simulink model "OFDM_RF_comms_link"  (R2023a)
settings: Solver=FixedStepAuto  StartTime=0.0  StopTime=Tstep*ofdmSymLen*6  RelTol=1e-3
PreLoadFcn:
  | % 100 MHz scenario
  | scs = 30e3;
  | fftLength = 4096;
  | NSubcarriers = 3276;
  | cpLength = 288;
  | windowLength = 20;
  | 
  | nGuardBandCarrier = fftLength - NSubcarriers;
  | ofdmSymLen = fftLength+cpLength;
  | overSamplingRate = 7;
  | filterLength = 6*70;
  | 
  | BW = scs*fftLength;                       %  Signal BW
  | Tstep = 1/BW;                   %  Simulation BW BB
  | RF = 3.7e9;                       %  RF center frequency
  | IF = 500e6;                          % IF frequency
  | dataRatePA = 1/BW;  % PA characterization sample time
  | N = nGuardBandCarrier/2;
  | HPF_cutoff = RF - 500e6;
  | 
  | bw = 100e6;
  | [txWaveform, sampleRate] = helperPACharGenerateOFDM(bw);
  | 
  | dataFileName = sprintf("helperPACharSavedData%dMHz",bw/1e6);
  | load(dataFileName,"results")
  | paInput = results.InputWaveform;
  | paOutput = results.OutputWaveform;
  | modType = 'memPoly';
  | memLen = 5;
  | degLen = 5;
  | halfDataPts = round(length(paInput)/2);
  | origState = warning;
  | warning('off', 'MATLAB:rankDeficientMatrix')
  | paModelMemPoly = double(helperPACharMemPolyModel('coefficientFinder', ...
  |   paInput(1:halfDataPts),paOutput(1:halfDataPts),memLen,degLen,modType));
  | warning(origState);
  | 
  | gain = results.LinearGain;
  | scaleFactor = double(max(abs(paOutput))/max(abs(txWaveform))/gain);
undefined symbols (not defined in the file or in its folder): QAM, rational, S, sparameters
libraries: simrfV2elements x17, simrfV2util1 x5, simrfV2_lib x3, commofdm x2, dspstat3 x2, commrfcorlib x2, commrandsrc3 x1, commdigbbndam3 x1, simrfV2junction1 x1, simrfV2sources1 x1, commutil2 x1, simrfV2systems x1
Description:
  | Power Amplifier Characterization with DPD for Reduced Signal Distortion
settings Model: SimulationMode=accelerator  Creator=The MathWorks, Inc.  LastModifiedBy=pradnyapatil
settings SolverCC: ZeroCrossAlgorithm=Adaptive  AlgebraicLoopSolver=TrustRegion
settings DataIOCC: LimitDataPoints=on  SaveFormat=Array  SaveOutput=off  SignalLogging=off  DSMLogging=off  SaveTime=off  ReturnWorkspaceOutputs=off
settings OptimizationCC: BlockReduction=off  BooleanDataType=off  ReuseModelBlockBuffer=off  LifeSpan=inf
settings DebuggingCC: SaveWithParameterizedLinksMsg=none  UnderspecifiedInitializationDetection=Classic  MergeDetectMultiDrivingBlocksExec=none  SignalResolutionControl=TryResolveAllWithWarning  UnconnectedInputMsg=warning  UnconnectedOutputMsg=warning  UnconnectedLineMsg=warning  AllowSymbolicDim=off  SFUnexpectedBacktrackingDiag=warning  SFNoUnconditionalDefaultTransitionDiag=warning  SFExecutionAtInitializationDiag=none  ArithmeticOperatorsInVariantConditions=warning
settings HardwareCC: ProdBitPerPointer=32  ProdBitPerSizeT=32  ProdBitPerPtrDiffT=32  ProdLargestAtomicFloat=None  ProdIntDivRoundTo=Undefined  ProdEndianess=Unspecified  ProdWordSize=32  ProdHWDeviceType=32-bit Generic  TargetBitPerLong=64  TargetBitPerPointer=64  TargetBitPerSizeT=64  TargetBitPerPtrDiffT=64  TargetLongLongMode=on  TargetIntDivRoundTo=Zero  TargetEndianess=LittleEndian  TargetWordSize=64  TargetHWDeviceType=MATLAB Host  ProdEqTarget=off
settings ModelReferenceCC: EnableRefExpFcnMdlSchedulingChecks=on  PropagateSignalLabelsOutOfModel=off
settings SFSimCC: SimUseLocalCustomCode=off
settings RTWCC: RTWUseLocalCustomCode=off  BuildConfiguration=Faster Runs  DLArmComputeVersion=19.05
settings CodeAppCC: StateflowObjectComments=on
settings GRTTargetCC: TargetLangStandard=C89/C90 (ANSI)
settings ConfigComp: CovMetricSettings=dw  CovSaveCumulativeToWorkspaceVar=on  CovSaveSingleToWorkspaceVar=on  CovExternalEMLEnable=off
settings SimscapeCC: SimscapeNormalizeSystem=off

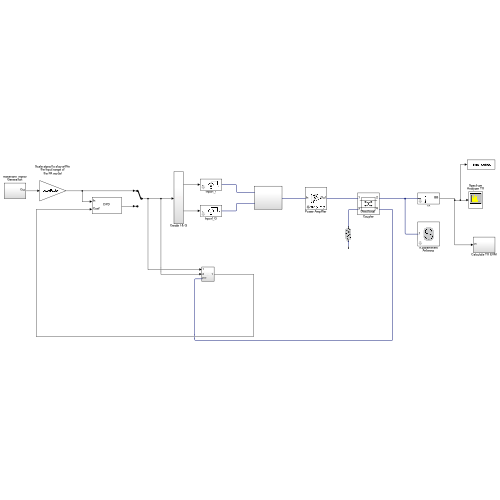
[thumbnail: Simulink's stored preview of the top-level diagram]
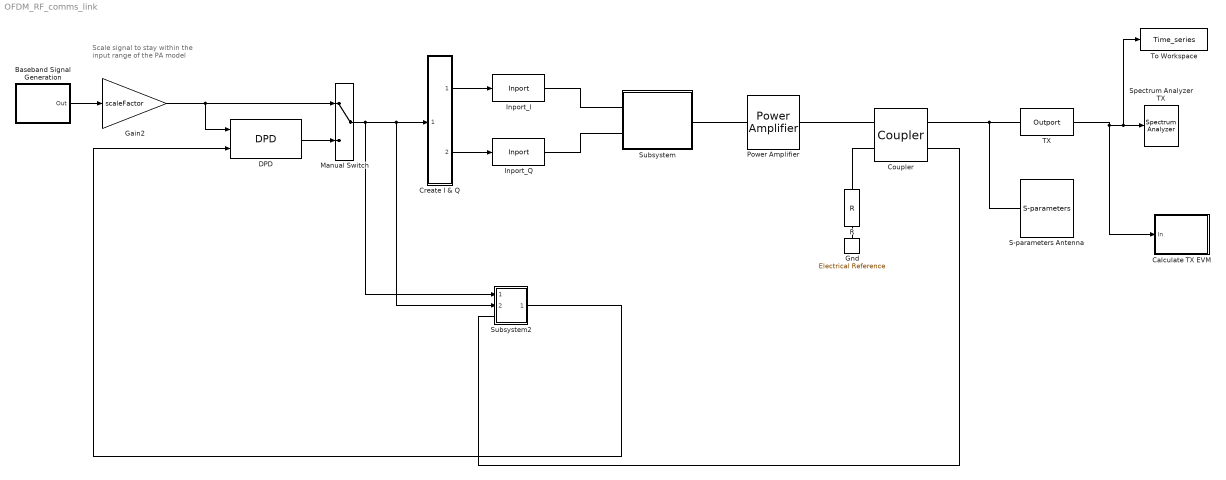
== system OFDM_RF_comms_link ==
  note: Scale signal to stay within
      | the input range of
      | the PA model
  Baseband Signal Generation : Subsystem
  Calculate TX EVM : Subsystem
  Coupler : simrfV2junction1/Coupler  classname=couplers  DataSource=Network-parameters  NumPorts=4  DeviceCirculator=Circulator clockwise  DeviceDivider=T power divider  DeviceCoupler=Directional coupler  Paramtype=S-parameters  Sparam=[0 0 1; 1 0 0; 0 1 0]  SparamFreq=1e9 Hz  SparamZ0=50  Phase12=0  Phase33=0  Alpha=0  NumberDividerOutports=2  Coupling=55  Directivity=inf  InsertionLoss=0.0001  ReturnLoss=inf  InternalGrounding=on  SparamRepresentation=Frequency domain  FitOpt=Share all poles  FitTol=-40  MaxPoles=48
  Create I & Q : Subsystem
  DPD : commrfcorlib/DPD  PolynomialType=Memory polynomial  CoefficientSource=Input port  Coefficients=complex([1 0 0 0 0; 0 0 0 0 0; 0 0 0 0 0])  SimulateUsing=Interpreted execution
  Gain2 : Gain  Gain=scaleFactor
  Gnd : simrfV2_lib/Elements/Electrical Reference
      settings: InternalSimscapePortConfiguration="{\"Bottom\":[],\"Left\":[{\"id\":\"V\",\"label\":\"\",\"type\":\"foundation.rf.circuitenvelope\"}],\"Right\":[],\"Top\":[]}"
  Inport_I : simrfV2util1/Inport  SimulinkInputSignalType=Ideal voltage  CarrierFreq=0 Hz  ZS=0  UseSqWave=off  NumCoeff=10  Bias=0  DutyCyc=50  InternalGrounding=on
  Inport_Q : simrfV2util1/Inport  SimulinkInputSignalType=Ideal voltage  CarrierFreq=0 Hz  ZS=0  UseSqWave=off  NumCoeff=10  Bias=0  DutyCyc=50  InternalGrounding=on
  Manual Switch : ManualSwitch
  Power Amplifier : simrfV2elements/Power Amplifier  classname=poweramp  ModelType=Memory polynomial  CoeffMatrix=paModelMemPoly  UnitDelay=dataRatePA/overSamplingRate  Rin=50  Rout=50  InternalGrounding=on
  R : simrfV2elements/R  classname=resistor  Resistance=50 Ohm  AddNoise=on
  S-parameters Antenna : simrfV2elements/S-parameters  classname=sparam_element  DataSource=Data file  File=antenna_dpdexample.s1p  isNetworkObj=off  NetworkObject=sparameters('default.s2p')  Paramtype=S-parameters  Sparam=[0 0;1 0]  SparamFreq=1e9 Hz  SparamZ0=50  isRationalObj=off  RationalObject=rational('default.s2p')  Residues=0  Poles=0  DF={0 0; 1 0}  FitOpt=Fit individually  FitTol=-40  MaxPoles=48  SourceFreq=Extracted from data source  PlotFreq=[1e9:1e6:3e9] Hz  PlotType=X-Y plane  YParam1=S(1,1)  YFormat1=Magnitude (dB)  YParam2=None  YFormat2=Magnitude (dB)  YOption=Linear  XOption=Linear  AddNoise=on  InternalGrounding=on  SparamRepresentation=Frequency domain  AutoImpulseLength=on  ImpulseLength=1e-10 s  MagModeling=off  CacheLevel=0
  Spectrum Analyzer TX : SpectrumAnalyzer  WindowPosition=[286.000000,108.000000,865.000000,471.000000,]  ScopeFrameLocation=window  Method=Welch  SampleRate=860160000  AxesScaling=Manual  Span=1843200000  StartFrequency=-921600000  StopFrequency=921600000  FrequencyResolutionMethod=Window length  WindowLength=8192  AveragingMethod=Running  SpectralAverages=4  ReferenceLoad=50  YLimits=[-42.635393903054115583 22.757787926364073883]  DefaultConfigurationName=spbscopes.SpectrumAnalyzerBlockCfg  IsFrequencyInputMode=0  FrequencyVectorPort=0  FrequencyVectorFromPort=0  FrequencyInputRBWPort=0  FrequencyInputRBWFromPort=0
  Subsystem : Subsystem
  Subsystem2 : Subsystem
  TX : simrfV2util1/Outport  SensorType=Ideal voltage  OutputFormat=Complex Baseband  CarrierFreq=RF Hz  ZL=Inf  InternalGrounding=on  StepSize=-1 s  AutoStep=off  HalfPolyphaseLength=0
  To Workspace : ToWorkspace  VariableName=Time_series  SaveFormat=Timeseries  SampleTime=-1
  wires:
  DPD/1 -> Manual Switch/2
  Create I & Q/1(Out1) -> Inport_I/1
  Create I & Q/2(Out2) -> Inport_Q/1
  Baseband Signal Generation/1(Out) -> Gain2/1
  Manual Switch/1 -> Subsystem2/1(In1), Subsystem2/2(In2), Create I & Q/1(In1)
  Gain2/1 -> DPD/1, Manual Switch/1
  TX/1 -> Calculate TX EVM/1(In), To Workspace/1, Spectrum Analyzer TX/1
  Subsystem2/1(Out1) -> DPD/2
  connections:
  S-parameters Antenna/LConn1 -- TX/LConn1 -- Coupler/RConn1
  Power Amplifier/RConn1 -- Coupler/LConn1
  R/LConn1 -- Coupler/LConn2
  Gnd/LConn1 -- R/RConn1
  Subsystem/LConn1 -- Inport_I/RConn1
  Power Amplifier/LConn1 -- Subsystem/RConn1
  Subsystem/LConn2 -- Inport_Q/RConn1
  Subsystem2/LConn1 -- Coupler/RConn2

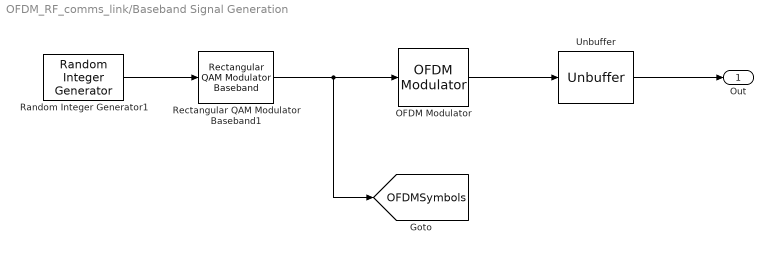
== system OFDM_RF_comms_link/Baseband Signal Generation ==
  OFDM Modulator : commofdm/OFDM Modulator  FFTLength=fftLength  NumGuardBandCarriers=[N+1; N]  InsertDCNull=off  PilotInputPort=off  PilotCarrierIndices=[12; 26; 40; 54]  CyclicPrefixLength=cpLength  Windowing=on  WindowLength=windowLength  OversamplingFactor=overSamplingRate  NumSymbols=1  NumTransmitAntennas=1  SimulateUsing=Interpreted execution
  Random Integer Generator1 : commrandsrc3/Random Integer Generator  SetSize=64  SeedSource=Parameter  Seed=242  SampleTime=Tstep*(ofdmSymLen/(fftLength-2*N-1))  SamplesPerFrame=fftLength-2*N-1  OutputDataType=double  SimulateUsing=Interpreted execution
  Rectangular QAM Modulator Baseband1 : commdigbbndam3/Rectangular QAM Modulator Baseband  M=64  InType=Integer  Enc=Gray  Mapping=[0:15]  PowType=Min. distance between symbols  MinDist=2  AvgPow=1  PeakPow=1  Ph=0  outDtype=double  outWordLen=16  outUDDataType=sfix(16)  outFracLenMode=Best precision  outFracLen=15  outDataTypeStr=double  outLastDataTypeStr=double
  Unbuffer : Unbuffer
  Out : Outport  VectorParamsAs1DForOutWhenUnconnected=off
  tag scope: OFDMSymbols=global
  wires:
  Random Integer Generator1/1 -> Rectangular QAM Modulator Baseband1/1
  Unbuffer/1 -> Out/1
  Rectangular QAM Modulator Baseband1/1 -> [OFDMSymbols], OFDM Modulator/1
  OFDM Modulator/1 -> Unbuffer/1

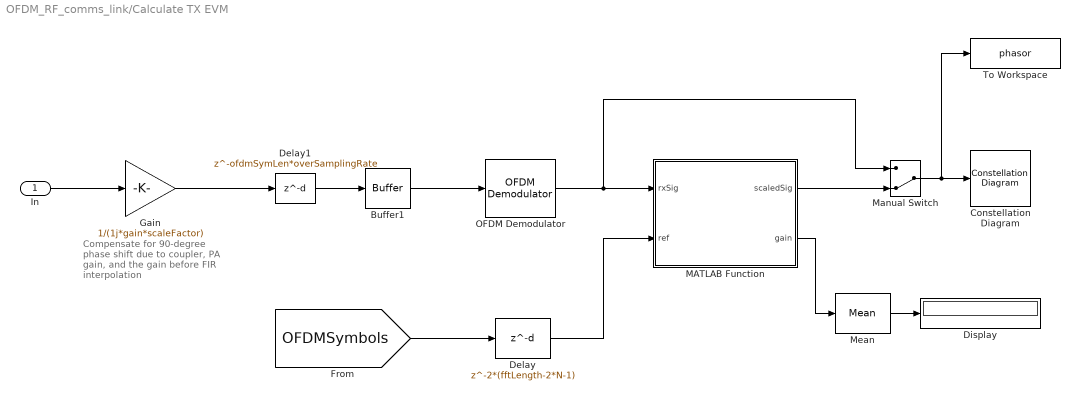
== system OFDM_RF_comms_link/Calculate TX EVM ==
  note: Compensate for 90-degree
      | phase shift due to coupler,
      | PA gain, and the gain before
      | FIR interpolation
  In : Inport
  Buffer1 : Buffer  N=ofdmSymLen*overSamplingRate  OutputFrames=off
  Constellation Diagram : ConstellationDiagram  WindowPosition=[467.000000,176.000000,612.000000,480.000000,]  ScopeFrameLocation=window  ReferenceConstellation=64-QAM  XLimits=[-9.7559 9.963]  YLimits=[-9.7559 9.963]  EnableMeasurements=on  DefaultConfigurationName=comm.scopes.ConstellationDiagramBlockCfg
  Delay : Delay  DelayLength=2*(fftLength-2*N-1)  InputProcessing=Columns as channels (frame based)
  Delay1 : Delay  DelayLength=ofdmSymLen*overSamplingRate  InputProcessing=Columns as channels (frame based)
  Display : Display
  Gain : Gain  Gain=1/(1j*gain*scaleFactor)
  MATLAB Function : MATLAB Function  TreatAsAtomicUnit=on
  Manual Switch : ManualSwitch  CurrentSetting=0
  Mean : dspstat3/Mean  run=off  InputProcessing=Columns as channels (frame based)  reset_popup=None  directionMode=Each column  dimension=1  roiEnable=off  roiType=Rectangles  roiPortion=Entire ROI  roiOutput=Individual statistics for each ROI  roiFlag=off  roundingMode=Floor  overflowMode=off  outputDataTypeStr=Inherit: Same as accumulator  outputMin=[]  outputMax=[]  outputLastDataTypeStr=Inherit: Same as accumulator
  OFDM Demodulator : commofdm/OFDM Demodulator  FFTLength=fftLength  NumGuardBandCarriers=[N+1; N]  RemoveDCCarrier=off  PilotOutputPort=off  PilotCarrierIndices=[12; 26; 40; 54]  CyclicPrefixLength=cpLength  OversamplingFactor=overSamplingRate  NumSymbols=1  NumReceiveAntennas=1  SimulateUsing=Interpreted execution
  To Workspace : ToWorkspace  VariableName=phasor  SaveFormat=Timeseries  SampleTime=-1
  wires:
  Buffer1/1 -> OFDM Demodulator/1
  In/1 -> Gain/1
  MATLAB Function/2(gain) -> Mean/1
  MATLAB Function/1(scaledSig) -> Manual Switch/2
  Manual Switch/1 -> To Workspace/1, Constellation Diagram/1
  OFDM Demodulator/1 -> MATLAB Function/1(rxSig), Manual Switch/1
  [OFDMSymbols] -> Delay/1
  Delay/1 -> MATLAB Function/2(ref)
  Mean/1 -> Display/1
  Gain/1 -> Delay1/1
  Delay1/1 -> Buffer1/1

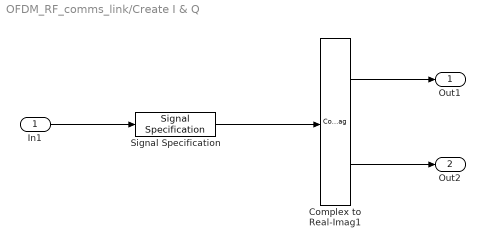
== system OFDM_RF_comms_link/Create I & Q ==
  In1 : Inport
  Complex to Real-Imag1 : ComplexToRealImag
  Signal Specification : SignalSpecification  Dimensions=1
  Out1 : Outport  VectorParamsAs1DForOutWhenUnconnected=off
  Out2 : Outport  Port=2  VectorParamsAs1DForOutWhenUnconnected=off
  wires:
  Complex to Real-Imag1/1 -> Out1/1
  Complex to Real-Imag1/2 -> Out2/1
  In1/1 -> Signal Specification/1
  Signal Specification/1 -> Complex to Real-Imag1/1

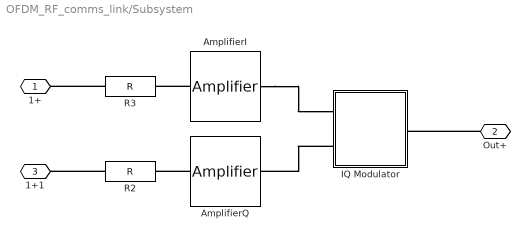
== system OFDM_RF_comms_link/Subsystem ==
  AmplifierI : simrfV2elements/Amplifier  classname=amplifier  DataSource=Data file  File=unitygain.s2p  isNetworkObj=off  Paramtype=S-parameters  Sparam=[0 0;1 0]  SparamFreq=1e9 Hz  SparamZ0=50  isRationalObj=off  Residues=0  Poles=0  DF={0 0; 1 0}  Source_linear_gain=Available power gain  linear_gain=10*log10(4) dB  AmAmAmPmTable=[-25,5,-1;-10,20,-2;0,27,5;5,28,12]  Zin=50  Zout=50  Source_Poly=Even and odd order  Poly_Coeffs=[0 1]  IPType=Input  IP2=inf dBm  IP3=inf dBm  P1dB=inf dBm  Psat=inf dBm  Gcomp=inf dBm  InternalGrounding=on  SourceFreq=Extracted from data source  PlotFreq=[1e9:1e6:3e9] Hz  PlotType=X-Y plane  YParam1=S(1,1)  YFormat1=Magnitude (dB)  YParam2=None  YFormat2=Magnitude (dB)  YOption=Linear  XOption=Linear  SparamRepresentation=Time domain (rationalfit)  FitTol=-40  FitOpt=Fit individually  MaxPoles=48  AutoImpulseLength=on  ImpulseLength=1e-10 s  MagModeling=off  AddNoise=on  NoiseType=Noise figure  NoiseDist=White  NF=amp_noise  MinNF=0  Gopt=0  RN=0  CarrierFreq=0 Hz  NoiseAutoImpulseLength=on  NoiseImpulseLength=1e-10 s  ConstS21NL=on  OpFreq=0 Hz  SetOpFreqAsMaxS21=on
  AmplifierQ : simrfV2elements/Amplifier  classname=amplifier  DataSource=Data file  File=unitygain.s2p  isNetworkObj=off  Paramtype=S-parameters  Sparam=[0 0;1 0]  SparamFreq=1e9 Hz  SparamZ0=50  isRationalObj=off  Residues=0  Poles=0  DF={0 0; 1 0}  Source_linear_gain=Available power gain  linear_gain=10*log10(4) dB  AmAmAmPmTable=[-25,5,-1;-10,20,-2;0,27,5;5,28,12]  Zin=50  Zout=50  Source_Poly=Even and odd order  Poly_Coeffs=[0 1]  IPType=Input  IP2=inf dBm  IP3=inf dBm  P1dB=inf dBm  Psat=inf dBm  Gcomp=inf dBm  InternalGrounding=on  SourceFreq=Extracted from data source  PlotFreq=[1e9:1e6:3e9] Hz  PlotType=X-Y plane  YParam1=S(1,1)  YFormat1=Magnitude (dB)  YParam2=None  YFormat2=Magnitude (dB)  YOption=Linear  XOption=Linear  SparamRepresentation=Time domain (rationalfit)  FitTol=-40  FitOpt=Fit individually  MaxPoles=48  AutoImpulseLength=on  ImpulseLength=1e-10 s  MagModeling=off  AddNoise=on  NoiseType=Noise figure  NoiseDist=White  NF=amp_noise  MinNF=0  Gopt=0  RN=0  CarrierFreq=0 Hz  NoiseAutoImpulseLength=on  NoiseImpulseLength=1e-10 s  ConstS21NL=on  OpFreq=0 Hz  SetOpFreqAsMaxS21=on
  IQ Modulator : Subsystem  DialogController=simrfV2DDGCreate
      settings: LibrarySourceBlock=simrfV2systems/IQ Modulator
      mask Display:
      | port_label('LConn', 1,'I')
      | port_label('LConn', 2,'Q')
      | port_label('RConn', 1,'Out')
  R2 : simrfV2elements/R  classname=resistor  Resistance=50 Ohm  AddNoise=on
  R3 : simrfV2elements/R  classname=resistor  Resistance=50 Ohm  AddNoise=on
  1+ : PMIOPort  Side=Left
  Out+ : PMIOPort  Port=2  Side=Right
  1+1 : PMIOPort  Port=3  Side=Left
  connections:
  Out+/RConn1 -- IQ Modulator/RConn1
  IQ Modulator/LConn2 -- AmplifierQ/RConn1
  AmplifierI/LConn1 -- R3/RConn1
  AmplifierI/RConn1 -- IQ Modulator/LConn1
  R3/LConn1 -- 1+/RConn1
  AmplifierQ/LConn1 -- R2/RConn1
  R2/LConn1 -- 1+1/RConn1

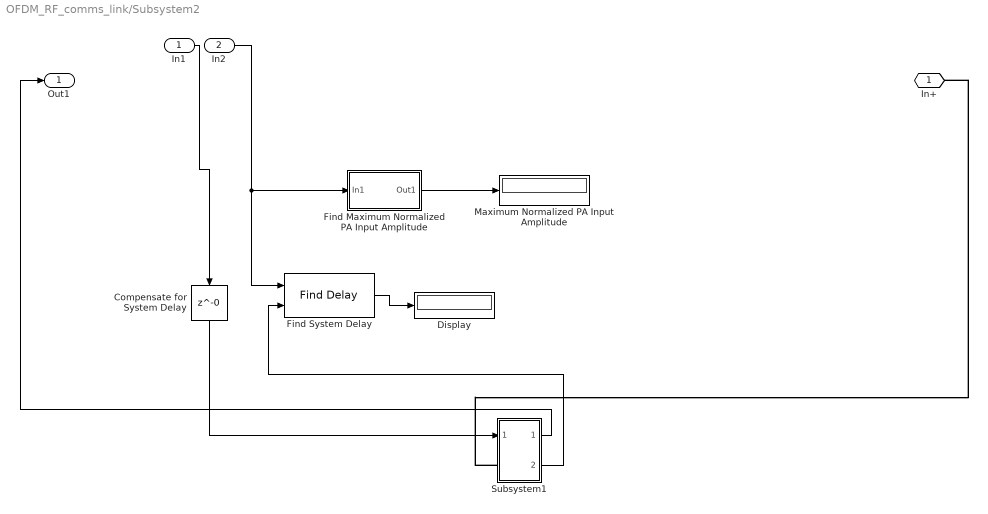
== system OFDM_RF_comms_link/Subsystem2 ==
  In1 : Inport
  In2 : Inport  Port=2
  Compensate for System Delay : Delay  DelayLength=0
  Display : Display
  Find Maximum Normalized PA Input Amplitude : Subsystem
  Find System Delay : commutil2/Find Delay  corrLength=200  chgSigOP=off  stopUpdate=off  numConstDelay=3
  Maximum Normalized PA Input Amplitude : Display
  Subsystem1 : Subsystem
  In+ : PMIOPort  Side=Left
  Out1 : Outport
  wires:
  Subsystem1/1(Out1) -> Out1/1
  In1/1 -> Compensate for System Delay/1
  Compensate for System Delay/1 -> Subsystem1/1(In1)
  Find Maximum Normalized PA Input Amplitude/1(Out1) -> Maximum Normalized PA Input Amplitude/1
  Subsystem1/2(Out2) -> Find System Delay/2
  Find System Delay/1 -> Display/1
  In2/1 -> Find System Delay/1, Find Maximum Normalized PA Input Amplitude/1(In1)
  connections:
  Subsystem1/LConn1 -- In+/RConn1

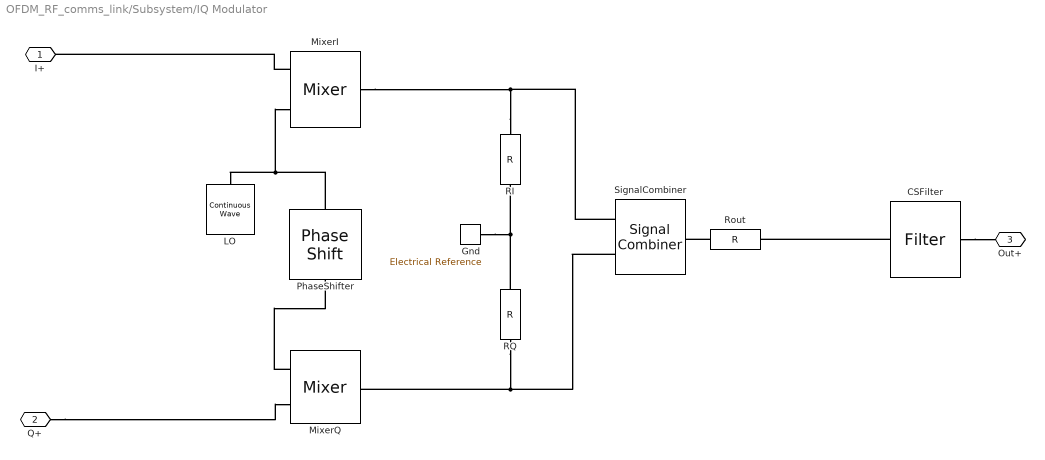
== system OFDM_RF_comms_link/Subsystem/IQ Modulator ==
  CSFilter : simrfV2elements/Filter  classname=filter  DesignMethod=Ideal  ResponseType=Highpass  Implementation=LC Tee  ImplementationIdeal=Constant per carrier  ImplementationRational=Transfer function  UseFilterOrder=on  FilterOrder=3  PassFreq_lp=1 GHz  PassFreq_hp=3200000000 Hz  PassFreq_bp=[2 3] GHz  PassFreq_bs=[1 4] GHz  PassAtten=3.01029995663981  StopFreq_lp=2 GHz  StopFreq_hp=1 GHz  StopFreq_bp=[1.5 3.5] GHz  StopFreq_bs=[2.1 2.9] GHz  StopAtten=40  Rsrc=50  Rload=50  AutoImpulseLength=on  ImpulseLength=1e-10 s  InternalGrounding=on  PlotFuncLeft=Voltage transfer  PlotLeftForm=Magnitude (dB)  PlotRightOnVT=None  PlotRightNoTD=None  PlotRightNoGD=None  PlotRightNoIR=None  PlotRightNoSR=None  PlotRightForm=Magnitude (dB)  FreqPoints=logspace(0,10,101)  Freq_unit=Hz  TimePoints=linspace(0,1,1e6+1)  Time_unit=s  XaxisScale=Linear  YaxisScale=Linear  needRedraw=1
  Gnd : simrfV2_lib/Elements/Electrical Reference
      settings: InternalSimscapePortConfiguration="{\"Bottom\":[],\"Left\":[{\"id\":\"V\",\"label\":\"\",\"type\":\"foundation.rf.circuitenvelope\"}],\"Right\":[],\"Top\":[]}"
  LO : simrfV2sources1/Continuous Wave  CWSourceType=Ideal voltage  Z0=0  IVoltage=1 V  ICurrent=0 A  MagPower=0 W  QVoltage=0 V  QCurrent=0 A  AnglePower=0  CarrierFreq=3700000000 Hz  AddPhaseNoise=off  PhaseNoiseOffset=1000000  PhaseNoiseLevel=-140  AutoImpulseLength=on  ImpulseLength=1e-10 s  InternalGrounding=on
  MixerI : simrfV2elements/Mixer  classname=mixer  Source_linear_gain=Available power gain  linear_gain=3.01029995663981 dB  Zin=50  Zout=50  ZLO=inf  Source_Poly=Even and odd order  Poly_Coeffs=[0 1]  IPType=Input  IP2=Inf dBm  IP3=Inf dBm  P1dB=Inf dBm  Psat=Inf dBm  Gcomp=Inf dBm  NF=0  InternalGrounding=on
  MixerQ : simrfV2elements/Mixer  classname=mixer  Source_linear_gain=Available power gain  linear_gain=3.01029995663981 dB  Zin=50  Zout=50  ZLO=inf  Source_Poly=Even and odd order  Poly_Coeffs=[0 1]  IPType=Input  IP2=Inf dBm  IP3=Inf dBm  P1dB=Inf dBm  Psat=Inf dBm  Gcomp=Inf dBm  NF=0  InternalGrounding=on
  PhaseShifter : simrfV2elements/Phase Shift  PhaseShift=90 deg  InternalGrounding=on
  RI : simrfV2elements/R  classname=resistor  Resistance=50 Ohm  AddNoise=off
  RQ : simrfV2elements/R  classname=resistor  Resistance=50 Ohm  AddNoise=off
  Rout : simrfV2elements/R  classname=resistor  Resistance=50 Ohm  AddNoise=off
  SignalCombiner : simrfV2elements/Signal Combiner  classname=signal_sum_mask  InternalGrounding=on
  I+ : PMIOPort  Side=Left
  Q+ : PMIOPort  Port=2  Side=Left
  Out+ : PMIOPort  Port=3  Side=Right
  connections:
  SignalCombiner/LConn2 -- RQ/LConn1 -- MixerQ/RConn1
  Rout/RConn1 -- SignalCombiner/RConn1
  Q+/RConn1 -- MixerQ/LConn1
  MixerI/LConn1 -- I+/RConn1
  RI/RConn1 -- Gnd/LConn1 -- RQ/RConn1
  CSFilter/LConn1 -- Rout/LConn1
  CSFilter/RConn1 -- Out+/RConn1
  MixerI/LConn2 -- PhaseShifter/LConn1 -- LO/LConn1
  RI/LConn1 -- MixerI/RConn1 -- SignalCombiner/LConn1
  MixerQ/LConn2 -- PhaseShifter/RConn1

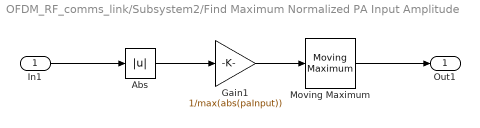
== system OFDM_RF_comms_link/Subsystem2/Find Maximum Normalized PA Input Amplitude ==
  In1 : Inport
  Abs : Abs  SaturateOnIntegerOverflow=off
  Gain1 : Gain  Gain=1/max(abs(paInput))
  Moving Maximum : dspstat3/Moving Maximum  SpecifyWindowLength=off  WindowLength=4  SimulateUsing=Interpreted execution
  Out1 : Outport
  wires:
  Abs/1 -> Gain1/1
  Gain1/1 -> Moving Maximum/1
  Moving Maximum/1 -> Out1/1
  In1/1 -> Abs/1

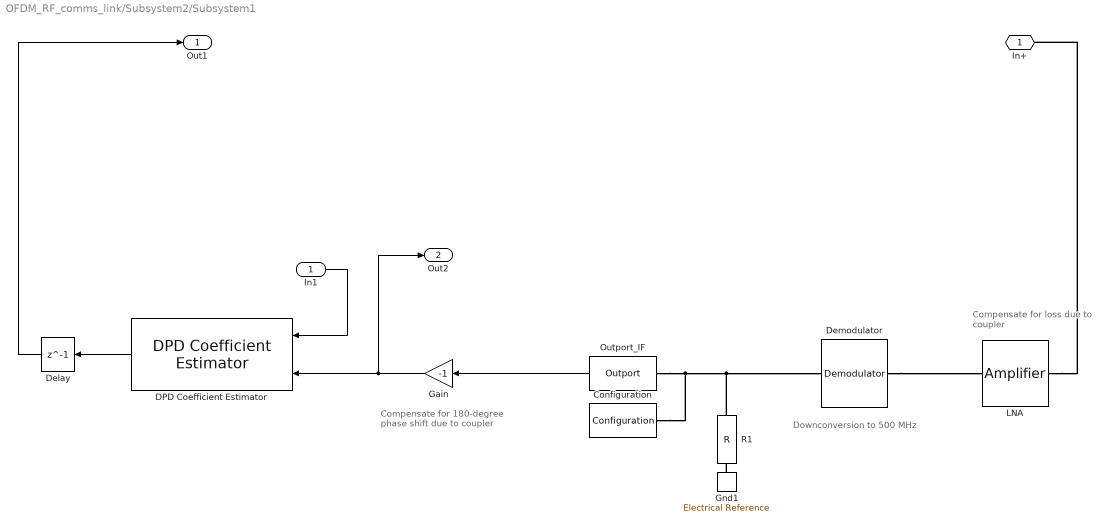
== system OFDM_RF_comms_link/Subsystem2/Subsystem1 ==
  note: Compensate for loss
      | due to coupler
  note: Compensate for 180-degree
      | phase shift due to coupler
  note: Downconversion
      | to 500 MHz
  In1 : Inport
  Configuration : simrfV2util1/Configuration  AutoFreq=on  Tones="[3.2         3.7] GHz"  Harmonics="[5  5]"  NormalizeCarrierPower=on  SolverType=Auto  UseCCode=on  StepSize=Tstep/overSamplingRate s  AddNoise=on  defaultRNG=on  Seed=0  Temperature=290.0 K  SolverDelFlag=0  AbsTol=1e-6  RelTol=1e-3  MaxIter=10  ErrorEstimationType=2-norm over all variables  EnableInterpFilter=off  HiddenFIRfilterControllerParam=off  SmallSignalApprox=off  AllSimFreqs=on  SimFreqs=[] Hz  SimFreqsInternal=[]  SamplesPerFrame=1
  DPD Coefficient Estimator : commrfcorlib/DPD Coefficient Estimator  DesiredAmplitudeGaindB=10*log10(gain)  PolynomialType=Memory polynomial  Degree=5  MemoryDepth=7  Algorithm=Recursive least squares  ForgettingFactorSource=Property  ForgettingFactor=0.9976  InitialCoefficientEstimate=[]  SimulateUsing=Interpreted execution
  Delay : Delay  DelayLength=1
  Demodulator : simrfV2systems/Demodulator  classname=rfdemod  Source_linear_gain=Available power gain  linear_gain=0 dB  Poly_Coeffs=[0 1]  LOFreq=RF-IF Hz  Zin=50  Zout=50  AddIRFilter=on  AddCSFilter=off  InternalGrounding=on  ForceNextInit=off  Source_Poly=Even and odd order  IPType=Input  IP2=inf dBm  IP3=inf dBm  P1dB=inf dBm  Psat=inf dBm  Gcomp=inf dBm  NF=1  Isolation=inf dB  AddPhaseNoise=off  PhaseNoiseOffset=[5e5 1e6 5e6]  PhaseNoiseLevel=[-108 -130 -140]  AutoImpulseLengthPN=on  ImpulseLengthPN=1e-10  ImpulseLength_unitPN=s  DesignMethodIR=Ideal  ResponseTypeIR=Highpass  ImplementationIR=LC Tee  ImplementationIdealIR=Constant per carrier  ImplementationRationalIR=Transfer function  UseFilterOrderIR=on  FilterOrderIR=3  PassFreq_lpIR=1  PassFreq_lp_unitIR=GHz  PassFreq_hpIR=HPF_cutoff  PassFreq_hp_unitIR=Hz  PassFreq_bpIR=[2 3]  PassFreq_bp_unitIR=GHz  PassFreq_bsIR=[1 4]  PassFreq_bs_unitIR=GHz  PassAttenIR=10*log10(2)  StopFreq_lpIR=2  StopFreq_lp_unitIR=GHz  StopFreq_hpIR=1  StopFreq_hp_unitIR=GHz  StopFreq_bpIR=[1.5 3.5]  StopFreq_bp_unitIR=GHz  StopFreq_bsIR=[2.1 2.9]  StopFreq_bs_unitIR=GHz  StopAttenIR=40  RsrcIR=50  RloadIR=50  AutoImpulseLengthIR=on  ImpulseLengthIR=1e-10  ImpulseLength_unitIR=s  DesignMethodCS=Ideal  ResponseTypeCS=Lowpass  ImplementationCS=LC Tee  ImplementationIdealCS=Constant per carrier  ImplementationRationalCS=Transfer function  UseFilterOrderCS=on  FilterOrderCS=3  PassFreq_lpCS=1  PassFreq_lp_unitCS=GHz  PassFreq_hpCS=2  PassFreq_hp_unitCS=GHz  PassFreq_bpCS=[2 3]  PassFreq_bp_unitCS=GHz  PassFreq_bsCS=[1 4]  PassFreq_bs_unitCS=GHz  PassAttenCS=10*log10(2)  StopFreq_lpCS=2  StopFreq_lp_unitCS=GHz  StopFreq_hpCS=1  StopFreq_hp_unitCS=GHz  StopFreq_bpCS=[1.5 3.5]  StopFreq_bp_unitCS=GHz  StopFreq_bsCS=[2.1 2.9]  StopFreq_bs_unitCS=GHz  StopAttenCS=40  RsrcCS=50  RloadCS=50  AutoImpulseLengthCS=on  ImpulseLengthCS=1e-10  ImpulseLength_unitCS=s
  Gain : Gain  Gain=-1
  Gnd1 : simrfV2_lib/Elements/Electrical Reference
      settings: InternalSimscapePortConfiguration="{\"Bottom\":[],\"Left\":[{\"id\":\"V\",\"label\":\"\",\"type\":\"foundation.rf.circuitenvelope\"}],\"Right\":[],\"Top\":[]}"
  LNA : simrfV2elements/Amplifier  classname=amplifier  DataSource=Data file  File=unitygain.s2p  isNetworkObj=off  Paramtype=S-parameters  Sparam=[0 0;1 0]  SparamFreq=1e9 Hz  SparamZ0=50  isRationalObj=off  Residues=0  Poles=0  DF={0 0; 1 0}  Source_linear_gain=Available power gain  linear_gain=55 dB  AmAmAmPmTable=[-25,5,-1;-10,20,-2;0,27,5;5,28,12]  Zin=50  Zout=50  Source_Poly=Odd order  Poly_Coeffs=[0 1]  IPType=Output  IP2=19.5 dBm  IP3=inf dBm  P1dB=inf dBm  Psat=inf dBm  Gcomp=inf dBm  InternalGrounding=on  SourceFreq=Extracted from data source  PlotFreq=0 Hz  PlotType=X-Y plane  YParam1=S(1,1)  YFormat1=Magnitude (dB)  YParam2=None  YFormat2=Magnitude (dB)  YOption=Linear  XOption=Linear  SparamRepresentation=Time domain (rationalfit)  FitTol=-40  FitOpt=Share all poles  MaxPoles=48  AutoImpulseLength=off  ImpulseLength=0 s  MagModeling=off  AddNoise=on  NoiseType=Noise figure  NoiseDist=White  NF=0.1  MinNF=0  Gopt=0  RN=0  CarrierFreq=0 Hz  NoiseAutoImpulseLength=on  NoiseImpulseLength=1e-10 s  ConstS21NL=on  OpFreq=0 Hz  SetOpFreqAsMaxS21=on
  Outport_IF : simrfV2util1/Outport  SensorType=Ideal voltage  OutputFormat=Complex Baseband  CarrierFreq=IF Hz  ZL=Inf  InternalGrounding=on  StepSize=-1 s  AutoStep=off  HalfPolyphaseLength=0
  R1 : simrfV2elements/R  classname=resistor  Resistance=50 Ohm  AddNoise=on
  In+ : PMIOPort  Side=Left
  Out1 : Outport
  Out2 : Outport  Port=2
  wires:
  DPD Coefficient Estimator/1 -> Delay/1
  Delay/1 -> Out1/1
  Outport_IF/1 -> Gain/1
  Gain/1 -> Out2/1, DPD Coefficient Estimator/2
  In1/1 -> DPD Coefficient Estimator/1
  connections:
  LNA/LConn1 -- In+/RConn1
  Outport_IF/LConn1 -- R1/LConn1 -- Demodulator/RConn1 -- Configuration/LConn1
  Demodulator/LConn1 -- LNA/RConn1
  Gnd1/LConn1 -- R1/RConn1

== matlab function OFDM_RF_comms_link/Calculate TX EVM/MATLAB Function ==
  data: rxSig input; scaledSig output; ref input; gain output
function [scaledSig, gain] = scaleRotate(rxSig,ref)
persistent c
persistent invCov
if isempty(c)
    c = complex(ones(size(rxSig)));
end
if isempty(invCov)
    invCov = complex(ones(size(rxSig)));
end

scaledSig = c.*rxSig;
errsig = ref - scaledSig;

% RLS algorithm
lambda = 0.99;
XP = conj(rxSig).*invCov;
invDen = 1./(lambda + XP.*rxSig);
K = invDen.*(invCov.*rxSig);
invCov = (1/lambda)*(invCov - K.*XP);
c = c + errsig .* conj(K);

gain = c;
